simulink model "CM13_2024a_MachE_for_UA_HIL"  (R2024a)
settings: Solver=ode1  StartTime=0.0  StopTime=Inf  FixedStep=0.001  RelTol=1e-3  EnableMultiTasking=on
PreLoadFcn:
  | % if ~length(which('cmcmd')), cmenv; end
PostLoadFcn:
  | if any(exist('dsrtsu_mdlpostloadfcn', 'file') ~= 0), dsrtsu_mdlpostloadfcn('Execute', bdroot); end
InitFcn:
  | , if any(exist('rtifpga_mdlclblib', 'file') ~= 0), rtifpga_mdlclblib('Init', bdroot); end,
  | , if any(exist('dsmpb_private', 'file') ~= 0), dsmpb_private('dsmpb_mdlclblib', 'Init', bdroot); end,
values from neighbouring files (symbols this model uses):
  CoastDown =     [Run_Simulink.mat]
  limitedMCT =     [Run_Simulink.mat]
  MCT =     [Run_Simulink.mat]
  pMCT =     [Run_Simulink.mat]
  RealSimPara =     [Run_Simulink.mat]
  Ref_speed = [13 13.007895099 13.015778396 13.023649891 13.031509584 13.039357475 13.047193564 13.055017851 13.062830336 13.070631019 13.0784199 13.086196979 ... (2669 elements, 2669x1)]    [Ref_speed_and_time.mat]
  Ref_time = [0 0.01 0.02 0.03 0.04 0.05 0.06 0.07 0.08 0.09 0.1 0.11 ... (2669 elements, 2669x1)]    [Ref_speed_and_time.mat]
  US06 =     [Run_Simulink.mat]
undefined symbols (not defined in the file or in its folder): AccelCmd, ActTqLF_Nm_, ActTqLR_Nm_, ActTqRF_Nm_, ActTqRR_Nm_, BattChargeLimitMaxPwr, BattChargeLimitSocBpts, BattChargeLimitTbl, BattChrgCapcty, BattDischargeLimitSocBpts, BattDischargeLimitTbl, BattDischargeMaxPwr, BattNumCellsParallel, BattNumCellsSeries, BattOpenVoltCapBpts, BattOpenVoltTbl, BattResistSocBpts, BattResistTbl, BattResistTempBpts, BrakeMaxPrs, BrakeMaxTrq, ChassisDistCg2FrontAxle, ChassisDistCg2RearAxle, ChassisVehMass, CltchCmd, DecelCmd, DiffRatio, DiscIntNeverNeededParam, EnvGravCnst, EnvPrs, EnvTemp, FuelSpecificGrav, GearCmd, h, InitStates, lgSw, MtrEffSpdBpts, MtrEffTbl, MtrEffTrqBpts, MtrPwrMax, MtrTrqMax, planned_speed, planned_time, ref_speed, ref_time, rticanmm_blockfcn, rticanmm_initfcn, SteeringCmd, SupvsryCtrlRegenBrkCutOffTbl, SupvsryCtrlRegenSpdBpts, TestScnrioCycleNum, VEH
libraries: simulink x264, VSIGenLib x262, etargetslib x201, dsmpblib x161, CarMaker4SL x142, rtimmsu_dsrtlib x32, vehdynlibtire x24, autolibshared x19, vehdynlibsuspension x14, vehdynlibtirecommon x14, autolibutils x10, VsrLibWheel x8
(part 2 of 48)

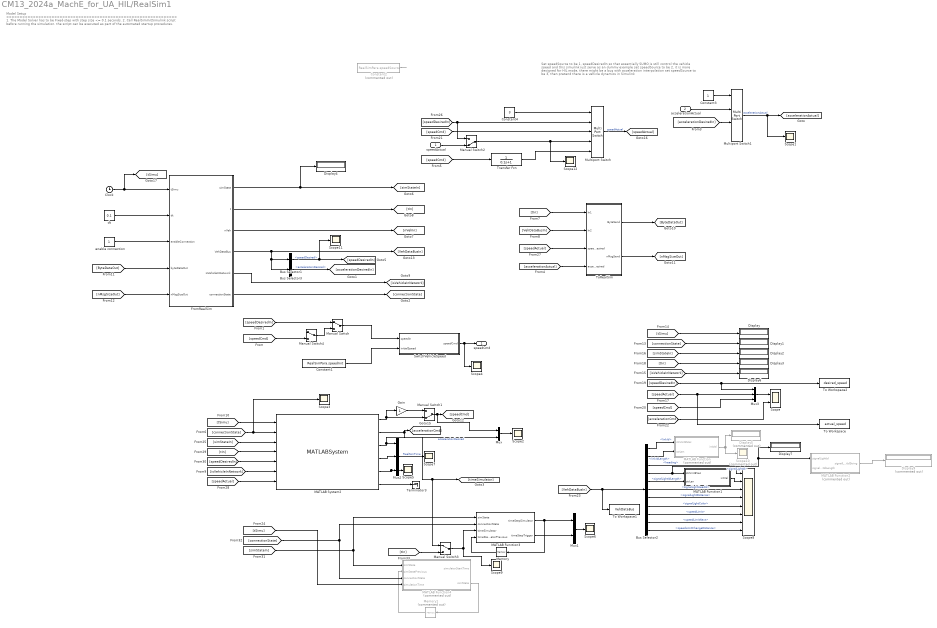
== system CM13_2024a_MachE_for_UA_HIL/RealSim1 ==
  note: Set speedSource to be 1, speedDesiredIn so that essentially SUMO is still control the vehicle speed and this simulink just serve as an dummy example
      |
      | set speedSource to be 2, it is more designed for HIL mode, there might be a bug with acceleration interpolation
      |
      | set speedSource to be 3, then pretend there is a vehicle dynamics in Simulink
  note: Model Setup
      | ================================================================
      | 1. The Model Solver has to be Fixed-step with step size <= 0.1 seconds.
      | 2. Call RealSimInitSimulink script before running the simulation. the script can be executed as part of the automated startup procedures.
  speedActual : Inport
  accelerationActual : Inport  Port=2
  Bus Selector1 : BusSelector  OutputSignals=speedDesired
  Bus Selector2 : BusSelector  OutputSignals=linkId,linkIdLength,heading,signalLightId,signalLightIdLength,signalLightHeadId,signalLightDistance,signalLightColor,speedLimit,speedLimitNext,speedLimitChangeDistance
  Bus Selector3 : BusSelector  OutputSignals=accelerationDesired
  Clock : Clock
  Constant1 : Constant  Value=RealSimPara.speedInit
  Constant2 : Constant  Commented=on  Value=RealSimPara.speedSource
  Constant3 : Constant
  Constant4 : Constant  Value=3
  Display{,1..4,6..7} (7 alike) : Display
  Display5 : Display  Commented=on
  Display9 : Display  Commented=on
  FromRealSim : Subsystem
  Gain : Gain
  MATLAB Function : MATLAB Function  Commented=on  TreatAsAtomicUnit=on
  MATLAB Function1 : MATLAB Function  TreatAsAtomicUnit=on
  MATLAB Function2 : MATLAB Function  Commented=on  TreatAsAtomicUnit=on  SystemSampleTime=0.001
  MATLAB Function3 : MATLAB Function  TreatAsAtomicUnit=on
  MATLAB Function4 : MATLAB Function  Commented=on  TreatAsAtomicUnit=on
  MATLAB System2 : MATLABSystem  System=RealSimInterpSpeed  initialSpeed=RealSimPara.speedInit  speedLookAheadHorizon=RealSimPara.tLookahead  speedUpperBound=30  smoothWindow=RealSimPara.smoothWindow  SimulateUsing=Interpreted execution
      mask Type: RealSimInterpSpeed
      mask Display:
      | disp('RealSimInterpSpeed');
      | port_label('input',1,'simulationTime');
      | port_label('input',2,'connectionState');
      | port_label('input',3,'simState');
      | port_label('input',4,'timeReceive');
      | port_label('input',5,'speedReceive');
      | port_label('input',6,'isVehicleInNetwork');
      | port_label('input',7,'speedActual');
      | port_label('output',1,'speedLookAhead');
      | port_label('output',2,'accelerationDesired');
      | port_label('output',3,'timeSimulator');
      | port_label('output',4,'timeStepSimulator');
      | port_label('output',5,'timeStepTrigger');
      | port_label('output',6,'RealSimDelay');
  Manual Switch : ManualSwitch
  Manual Switch1 : ManualSwitch  CurrentSetting=0
  Manual Switch2 : ManualSwitch  CurrentSetting=0
  Manual Switch3 : ManualSwitch
  Manual Switch4 : ManualSwitch
  Memory : Memory
  Memory1 : Memory  Commented=on
  Multiport Switch : MultiPortSwitch  Inputs=4  SaturateOnIntegerOverflow=off  InputSameDT=off
  Multiport Switch1 : MultiPortSwitch  SaturateOnIntegerOverflow=off  InputSameDT=off
  Mux : Mux  Inputs=2
  Mux1 : Mux  Inputs=2
  Mux2 : Mux  Inputs=3
  Mux3 : Mux  Inputs=3
  Scope : Scope  NumInputPorts=2
  Scope{1..7,9,11..12} (10 alike) : Scope
  Scope10 : Scope  Commented=on
  Scope8 : Scope  NumInputPorts=8
  SwitchVehicleSpeed : Subsystem
  Terminator3 : Terminator
  To Workspace : ToWorkspace  VariableName=actual_speed  SaveFormat=Timeseries  SampleTime=0.1
  To Workspace1 : ToWorkspace  VariableName=VehDataBus  SaveFormat=Timeseries  SampleTime=-1
  To Workspace2 : ToWorkspace  VariableName=desired_speed  SaveFormat=Timeseries  SampleTime=0.1
  ToRealSim : Subsystem
  Transfer Fcn : TransferFcn  Denominator=[0.1 1]
  dt : Constant  Value=0.1
  enable connection : Constant
  speedCmd : Outport
  wires:
  [speedCmd] -> Manual Switch4/2
  Manual Switch3/1 -> MATLAB Function3/3(timeSimulator), Scope9/1
  [tIn] -> Manual Switch3/2
  MATLAB Function4/2(simState) -> Memory1/1
  Memory1/1 -> MATLAB Function4/2(simStatePrevious)
  MATLAB Function3/2(timeStepTrigger) -> Mux1/2
  Mux1/1 -> Scope6/1
  Memory/1 -> MATLAB Function3/4(timeStepSimulatorPrevious)
  MATLAB Function3/1(timeStepSimulator) -> Memory/1, Mux1/1
  [simStateIn] -> MATLAB Function3/1(simState), MATLAB Function4/1("simState ")
  [connectionState] -> MATLAB Function3/2(connectionState), MATLAB Function4/3(connectionState)
  [tSimu] -> MATLAB Function4/4(simulationTime)
  Transfer Fcn/1 -> Multiport Switch/5
  [speedCmd] -> Transfer Fcn/1
  speedActual/1 -> Manual Switch2/2
  Mux/1 -> Scope2/1
  FromRealSim/6(connectionState) -> [connectionState]
  Multiport Switch1/1 -> [accelerationActual], Scope1/1  "accelerationActual"
  accelerationActual/1 -> Multiport Switch1/2
  [accelerationDesiredIn] -> Multiport Switch1/3
  Constant3/1 -> Multiport Switch1/1
  Bus Selector3/1 -> [accelerationDesiredIn]  "<accelerationDesired>"
  Manual Switch/1 -> SwitchVehicleSpeed/1(speedIn)
  SwitchVehicleSpeed/1(speedCmd) -> speedCmd/1, Scope4/1
  Constant1/1 -> SwitchVehicleSpeed/2(initialSpeed)
  [speedDesiredIn] -> Manual Switch/1
  Manual Switch4/1 -> Manual Switch/2
  Constant2/1 -> ?
  ? -> MATLAB Function2/2(signalLightIdLength)
  [simStateIn] -> Display2/1
  Mux3/1 -> Scope/1
  [isVehicleInNetwork] -> MATLAB System2/6
  Bus Selector2/3 -> Scope8/1  "<heading>"
  MATLAB Function1/1(intVal) -> Scope8/2
  ToRealSim/1(ByteSend) -> [ByteDataOut]
  [accelerationActual] -> ToRealSim/4(accelerationDesired)
  Bus Selector2/6 -> Scope8/3  "<signalLightHeadId>"
  Multiport Switch/1 -> [speedActual]  "speedActual"
  [VehDataBusIn] -> ToRealSim/2(In2)
  [accelerationCmd] -> Scope/2
  FromRealSim/5(isVehicleInNetwork) -> [isVehicleInNetwork]
  FromRealSim/2(t) -> [tIn]
  [speedActual] -> ToRealSim/3(speedDesired)
  FromRealSim/1(simState) -> [simStateIn], Display4/1
  ToRealSim/2(nMsgSend) -> [nMsgSizeOut]
  Manual Switch1/1 -> [speedCmd], Mux/1
  Constant4/1 -> Multiport Switch/1
  [speedCmd] -> Mux3/3
  [tIn] -> MATLAB System2/4
  Bus Selector2/2 -> MATLAB Function/2(strLen)  "<linkIdLength>"
  MATLAB Function2/1(signalLightIdString) -> Display9/1
  MATLAB System2/2 -> Mux/2, [accelerationCmd]  "accelerationDesired"
  [tIn] -> ToRealSim/1(In1)
  Bus Selector2/1 -> MATLAB Function/1(strUint8Vec)  "<linkId>"
  MATLAB System2/6 -> Terminator3/1
  [connectionState] -> Scope3/1, MATLAB System2/2
  Manual Switch2/1 -> Multiport Switch/4, Scope12/1
  Bus Selector2/8 -> Scope8/5  "<signalLightColor>"
  MATLAB System2/4 -> Mux2/2
  Bus Selector2/7 -> Scope8/4  "<signalLightDistance>"
  [tIn] -> Display3/1
  Clock/1 -> [tSimu], FromRealSim/1(tSimu)
  [connectionState] -> Display1/1
  [speedActual] -> Mux3/2, To Workspace/1
  FromRealSim/3(nVeh) -> [nVehIn]
  [speedActual] -> MATLAB System2/7
  [speedDesiredIn] -> Multiport Switch/2, Manual Switch2/1
  Bus Selector2/11 -> Scope8/8  "<speedLimitChangeDistance>"
  [nMsgSizeOut] -> FromRealSim/5(nMsgSizeOut)
  [speedDesiredIn] -> MATLAB System2/5
  MATLAB Function/1(intVal) -> Display5/1, Scope10/1
  enable connection/1 -> FromRealSim/3(enableConnection)
  FromRealSim/4(VehDataBus) -> Bus Selector3/1, Bus Selector1/1, [VehDataBusIn]
  Bus Selector2/10 -> Scope8/7  "<speedLimitNext>"
  dt/1 -> FromRealSim/2(dt)
  MATLAB System2/3 -> Mux2/1, Manual Switch3/1, [timeSimulator]
  Bus Selector2/4 -> MATLAB Function1/1(strUint8Vec), MATLAB Function2/1(signalLightId), Display7/1  "<signalLightId>"
  [speedDesiredIn] -> Mux3/1, To Workspace2/1
  Bus Selector2/9 -> Scope8/6  "<speedLimit>"
  Bus Selector1/1 -> [speedDesiredIn], Scope11/1  "<speedDesired>"
  Gain/1 -> Manual Switch1/1
  [tSimu] -> MATLAB System2/1
  Mux2/1 -> Scope7/1  "RealSimTime"
  [speedCmd] -> Multiport Switch/3
  MATLAB System2/1 -> Manual Switch1/2, Gain/1
  [VehDataBusIn] -> Bus Selector2/1, To Workspace1/1
  MATLAB System2/5 -> Mux2/3, Scope5/1
  [ByteDataOut] -> FromRealSim/4(byteDataOut)
  [isVehicleInNetwork] -> Display6/1
  [simStateIn] -> MATLAB System2/3
  Bus Selector2/5 -> MATLAB Function1/2(strLen)  "<signalLightIdLength>"
  [tSimu] -> Display/1

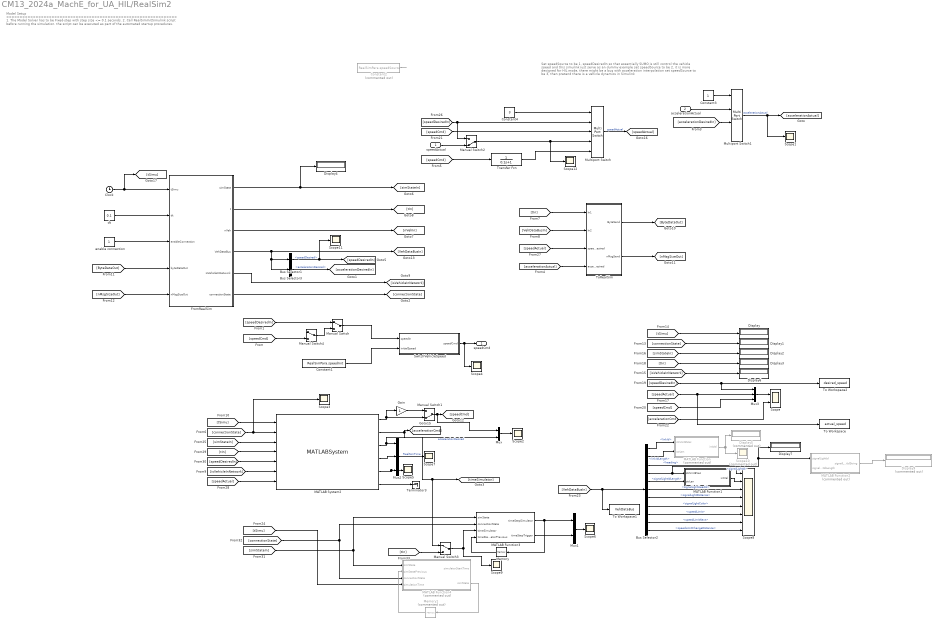
== system CM13_2024a_MachE_for_UA_HIL/RealSim2 ==
  note: Model Setup
      | ================================================================
      | 1. The Model Solver has to be Fixed-step with step size <= 0.1 seconds.
      | 2. Call RealSimInitSimulink script before running the simulation. the script can be executed as part of the automated startup procedures.
  note: Set speedSource to be 1, speedDesiredIn so that essentially SUMO is still control the vehicle speed and this simulink just serve as an dummy example
      |
      | set speedSource to be 2, it is more designed for HIL mode, there might be a bug with acceleration interpolation
      |
      | set speedSource to be 3, then pretend there is a vehicle dynamics in Simulink
  speedActual : Inport
  accelerationActual : Inport  Port=2
  Bus Selector1 : BusSelector  OutputSignals=speedDesired
  Bus Selector2 : BusSelector  OutputSignals=linkId,linkIdLength,heading,signalLightId,signalLightIdLength,signalLightHeadId,signalLightDistance,signalLightColor,speedLimit,speedLimitNext,speedLimitChangeDistance
  Bus Selector3 : BusSelector  OutputSignals=accelerationDesired
  Clock : Clock
  Constant1 : Constant  Value=RealSimPara.speedInit
  Constant2 : Constant  Commented=on  Value=RealSimPara.speedSource
  Constant3 : Constant
  Constant4 : Constant  Value=3
  Display{,1..4,6..7} (7 alike) : Display
  Display5 : Display  Commented=on
  Display9 : Display  Commented=on
  FromRealSim : Subsystem
  Gain : Gain
  MATLAB Function : MATLAB Function  Commented=on  TreatAsAtomicUnit=on
  MATLAB Function1 : MATLAB Function  TreatAsAtomicUnit=on
  MATLAB Function2 : MATLAB Function  Commented=on  TreatAsAtomicUnit=on  SystemSampleTime=0.001
  MATLAB Function3 : MATLAB Function  TreatAsAtomicUnit=on
  MATLAB Function4 : MATLAB Function  Commented=on  TreatAsAtomicUnit=on
  MATLAB System2 : MATLABSystem  System=RealSimInterpSpeed  initialSpeed=RealSimPara.speedInit  speedLookAheadHorizon=RealSimPara.tLookahead  speedUpperBound=30  smoothWindow=RealSimPara.smoothWindow  SimulateUsing=Interpreted execution
      mask Type: RealSimInterpSpeed
      mask Display:
      | disp('RealSimInterpSpeed');
      | port_label('input',1,'simulationTime');
      | port_label('input',2,'connectionState');
      | port_label('input',3,'simState');
      | port_label('input',4,'timeReceive');
      | port_label('input',5,'speedReceive');
      | port_label('input',6,'isVehicleInNetwork');
      | port_label('input',7,'speedActual');
      | port_label('output',1,'speedLookAhead');
      | port_label('output',2,'accelerationDesired');
      | port_label('output',3,'timeSimulator');
      | port_label('output',4,'timeStepSimulator');
      | port_label('output',5,'timeStepTrigger');
      | port_label('output',6,'RealSimDelay');
  Manual Switch : ManualSwitch
  Manual Switch1 : ManualSwitch  CurrentSetting=0
  Manual Switch2 : ManualSwitch  CurrentSetting=0
  Manual Switch3 : ManualSwitch
  Manual Switch4 : ManualSwitch
  Memory : Memory
  Memory1 : Memory  Commented=on
  Multiport Switch : MultiPortSwitch  Inputs=4  SaturateOnIntegerOverflow=off  InputSameDT=off
  Multiport Switch1 : MultiPortSwitch  SaturateOnIntegerOverflow=off  InputSameDT=off
  Mux : Mux  Inputs=2
  Mux1 : Mux  Inputs=2
  Mux2 : Mux  Inputs=3
  Mux3 : Mux  Inputs=3
  Scope : Scope  NumInputPorts=2
  Scope{1..7,9,11..12} (10 alike) : Scope
  Scope10 : Scope  Commented=on
  Scope8 : Scope  NumInputPorts=8
  SwitchVehicleSpeed : Subsystem
  Terminator3 : Terminator
  To Workspace : ToWorkspace  VariableName=actual_speed  SaveFormat=Timeseries  SampleTime=0.1
  To Workspace1 : ToWorkspace  VariableName=VehDataBus  SaveFormat=Timeseries  SampleTime=-1
  To Workspace2 : ToWorkspace  VariableName=desired_speed  SaveFormat=Timeseries  SampleTime=0.1
  ToRealSim : Subsystem
  Transfer Fcn : TransferFcn  Denominator=[0.1 1]
  dt : Constant  Value=0.1
  enable connection : Constant
  speedCmd : Outport
  wires:
  [tSimu] -> Display/1
  Bus Selector2/5 -> MATLAB Function1/2(strLen)  "<signalLightIdLength>"
  [simStateIn] -> MATLAB System2/3
  [isVehicleInNetwork] -> Display6/1
  [ByteDataOut] -> FromRealSim/4(byteDataOut)
  MATLAB System2/5 -> Scope5/1, Mux2/3
  [VehDataBusIn] -> To Workspace1/1, Bus Selector2/1
  MATLAB System2/1 -> Gain/1, Manual Switch1/2
  [speedCmd] -> Multiport Switch/3
  Mux2/1 -> Scope7/1  "RealSimTime"
  [tSimu] -> MATLAB System2/1
  Gain/1 -> Manual Switch1/1
  Bus Selector1/1 -> Scope11/1, [speedDesiredIn]  "<speedDesired>"
  Bus Selector2/9 -> Scope8/6  "<speedLimit>"
  [speedDesiredIn] -> To Workspace2/1, Mux3/1
  Bus Selector2/4 -> Display7/1, MATLAB Function2/1(signalLightId), MATLAB Function1/1(strUint8Vec)  "<signalLightId>"
  MATLAB System2/3 -> [timeSimulator], Manual Switch3/1, Mux2/1
  dt/1 -> FromRealSim/2(dt)
  Bus Selector2/10 -> Scope8/7  "<speedLimitNext>"
  FromRealSim/4(VehDataBus) -> [VehDataBusIn], Bus Selector1/1, Bus Selector3/1
  enable connection/1 -> FromRealSim/3(enableConnection)
  MATLAB Function/1(intVal) -> Scope10/1, Display5/1
  [speedDesiredIn] -> MATLAB System2/5
  [nMsgSizeOut] -> FromRealSim/5(nMsgSizeOut)
  Bus Selector2/11 -> Scope8/8  "<speedLimitChangeDistance>"
  [speedDesiredIn] -> Manual Switch2/1, Multiport Switch/2
  [speedActual] -> MATLAB System2/7
  FromRealSim/3(nVeh) -> [nVehIn]
  [speedActual] -> To Workspace/1, Mux3/2
  [connectionState] -> Display1/1
  Clock/1 -> FromRealSim/1(tSimu), [tSimu]
  [tIn] -> Display3/1
  Bus Selector2/7 -> Scope8/4  "<signalLightDistance>"
  MATLAB System2/4 -> Mux2/2
  Bus Selector2/8 -> Scope8/5  "<signalLightColor>"
  Manual Switch2/1 -> Scope12/1, Multiport Switch/4
  [connectionState] -> MATLAB System2/2, Scope3/1
  MATLAB System2/6 -> Terminator3/1
  Bus Selector2/1 -> MATLAB Function/1(strUint8Vec)  "<linkId>"
  [tIn] -> ToRealSim/1(In1)
  MATLAB System2/2 -> [accelerationCmd], Mux/2  "accelerationDesired"
  MATLAB Function2/1(signalLightIdString) -> Display9/1
  Bus Selector2/2 -> MATLAB Function/2(strLen)  "<linkIdLength>"
  [tIn] -> MATLAB System2/4
  [speedCmd] -> Mux3/3
  Constant4/1 -> Multiport Switch/1
  Manual Switch1/1 -> Mux/1, [speedCmd]
  ToRealSim/2(nMsgSend) -> [nMsgSizeOut]
  FromRealSim/1(simState) -> Display4/1, [simStateIn]
  [speedActual] -> ToRealSim/3(speedDesired)
  FromRealSim/2(t) -> [tIn]
  FromRealSim/5(isVehicleInNetwork) -> [isVehicleInNetwork]
  [accelerationCmd] -> Scope/2
  [VehDataBusIn] -> ToRealSim/2(In2)
  Multiport Switch/1 -> [speedActual]  "speedActual"
  Bus Selector2/6 -> Scope8/3  "<signalLightHeadId>"
  [accelerationActual] -> ToRealSim/4(accelerationDesired)
  ToRealSim/1(ByteSend) -> [ByteDataOut]
  MATLAB Function1/1(intVal) -> Scope8/2
  Bus Selector2/3 -> Scope8/1  "<heading>"
  [isVehicleInNetwork] -> MATLAB System2/6
  Mux3/1 -> Scope/1
  [simStateIn] -> Display2/1
  ? -> MATLAB Function2/2(signalLightIdLength)
  Constant2/1 -> ?
  Manual Switch4/1 -> Manual Switch/2
  [speedDesiredIn] -> Manual Switch/1
  Constant1/1 -> SwitchVehicleSpeed/2(initialSpeed)
  SwitchVehicleSpeed/1(speedCmd) -> Scope4/1, speedCmd/1
  Manual Switch/1 -> SwitchVehicleSpeed/1(speedIn)
  Bus Selector3/1 -> [accelerationDesiredIn]  "<accelerationDesired>"
  Constant3/1 -> Multiport Switch1/1
  [accelerationDesiredIn] -> Multiport Switch1/3
  accelerationActual/1 -> Multiport Switch1/2
  Multiport Switch1/1 -> Scope1/1, [accelerationActual]  "accelerationActual"
  FromRealSim/6(connectionState) -> [connectionState]
  Mux/1 -> Scope2/1
  speedActual/1 -> Manual Switch2/2
  [speedCmd] -> Transfer Fcn/1
  Transfer Fcn/1 -> Multiport Switch/5
  [tSimu] -> MATLAB Function4/4(simulationTime)
  [connectionState] -> MATLAB Function4/3(connectionState), MATLAB Function3/2(connectionState)
  [simStateIn] -> MATLAB Function4/1("simState "), MATLAB Function3/1(simState)
  MATLAB Function3/1(timeStepSimulator) -> Mux1/1, Memory/1
  Memory/1 -> MATLAB Function3/4(timeStepSimulatorPrevious)
  Mux1/1 -> Scope6/1
  MATLAB Function3/2(timeStepTrigger) -> Mux1/2
  Memory1/1 -> MATLAB Function4/2(simStatePrevious)
  MATLAB Function4/2(simState) -> Memory1/1
  [tIn] -> Manual Switch3/2
  Manual Switch3/1 -> Scope9/1, MATLAB Function3/3(timeSimulator)
  [speedCmd] -> Manual Switch4/2

== system CM13_2024a_MachE_for_UA_HIL/TCP SCALEXIO ==
  note: Receiving gas, brake, steering; or three identical speeds
  note: Sending out x, y, heading, time, and speed
  VehOutput : Inport
  comm : Inport  Port=2
  Constant2 : Constant  Value=zeros(1004,1);  OutDataTypeStr=uint8
  Data Type Conversion1 : DataTypeConversion  OutDataTypeStr=double  SaturateOnIntegerOverflow=off  RndMeth=Floor
  Data Type Conversion2 : DataTypeConversion  SaturateOnIntegerOverflow=off  RndMeth=Floor
  Data Type Conversion3 : DataTypeConversion  OutDataTypeStr=boolean  SaturateOnIntegerOverflow=off  RndMeth=Floor
  Defloater{,1..4} (5 alike) : VSIGenLib/Defloater  SystemSampleTime=-1  VariantActivationTime=update diagram  AllowFlexibleInterface=on  Latency=0  AutoFrameSizeCalculation=off
  Demux{,2..5} (5 alike) : Demux
  Demux1 : Demux  Outputs=5
  Display3 : Display
  Ethernet Setup Carla : dsmpblib/Data Inport  Priority=10000
      settings: SourceProductName=dSPACE Model Interface Package for Simulink (MIPS)
  Floater : VSIGenLib/Floater  SystemSampleTime=-1  VariantActivationTime=update diagram  AllowFlexibleInterface=on  Latency=0  AutoFrameSizeCalculation=off
  Floater1 : VSIGenLib/Floater  SystemSampleTime=-1  VariantActivationTime=update diagram  AllowFlexibleInterface=on  Latency=0  AutoFrameSizeCalculation=off
  Floater2 : VSIGenLib/Floater  SystemSampleTime=-1  VariantActivationTime=update diagram  AllowFlexibleInterface=on  Latency=0  AutoFrameSizeCalculation=off
  Mux : Mux  Inputs=21
  Mux1 : Mux  Inputs=3
  Receive [TCP Carla] : dsmpblib/Data Inport  Priority=10000
      settings: SourceProductName=dSPACE Model Interface Package for Simulink (MIPS)
  Scope1 : Scope
  Scope4 : Scope
  Selector1 : Selector  InputPortWidth=1024  IndexOptions=Index vector (dialog)  Indices=[8 7 6 5]  OutputSizes=1
  Selector2 : Selector  InputPortWidth=1024  IndexOptions=Index vector (dialog)  Indices=[12 11 10 9]  OutputSizes=1
  Selector4 : Selector  InputPortWidth=1024  IndexOptions=Index vector (dialog)  Indices=[4 3 2 1]  OutputSizes=1
  SpdAdjust : Gain  Gain=1.1414
  Status/Control_In [TCP Carla] : dsmpblib/Data Inport  Priority=10000
      settings: SourceProductName=dSPACE Model Interface Package for Simulink (MIPS)
  Status/Control_Out [TCP Carla] : dsmpblib/Data Outport  Priority=-10000
      settings: SourceProductName=dSPACE Model Interface Package for Simulink (MIPS)
  Terminator{1..5} (5 alike) : Terminator
  Transmit_In [TCP Carla] : dsmpblib/Data Inport  Priority=10000
      settings: SourceProductName=dSPACE Model Interface Package for Simulink (MIPS)
  Transmit_Out [TCP Carla] : dsmpblib/Data Outport  Priority=-10000
      settings: SourceProductName=dSPACE Model Interface Package for Simulink (MIPS)
  uint8 (unsigned 8) 4 : etargetslib/Byte Pack  datatypes={'uint8'}  byteAlign=1
  Output : Outport
  wires:
  Demux4/4 -> Mux/16
  Demux3/4 -> Mux/12
  Defloater1/1 -> Demux2/1
  Mux/1 -> Data Type Conversion2/1
  Demux4/2 -> Mux/14
  Demux3/1 -> Mux/9
  Demux/4 -> Mux/4
  Demux/1 -> Mux/1
  Demux2/4 -> Mux/8
  Demux1/3 -> Defloater2/1
  Defloater/1 -> Demux/1
  Defloater3/1 -> Demux4/1
  Demux3/3 -> Mux/11
  Demux1/2 -> Defloater1/1
  Demux2/2 -> Mux/6
  Constant2/1 -> uint8 (unsigned 8) 4/1
  Demux1/1 -> Defloater/1
  Defloater2/1 -> Demux3/1
  Demux1/4 -> Defloater3/1
  Demux3/2 -> Mux/10
  Demux/3 -> Mux/3
  Demux/2 -> Mux/2
  VehOutput/1 -> Demux1/1
  Demux2/1 -> Mux/5
  Demux4/1 -> Mux/13
  Demux2/3 -> Mux/7
  Demux4/3 -> Mux/15
  Data Type Conversion2/1 -> Transmit_Out [TCP Carla]/1
  ? -> Terminator2/1
  Transmit_In [TCP Carla]/1 -> Terminator1/1
  Receive [TCP Carla]/1 -> Selector2/1, Selector1/1, Selector4/1
  Selector4/1 -> Floater/1
  Floater/1 -> Display3/1, Mux1/1
  ? -> Terminator4/1
  Data Type Conversion3/1 -> Status/Control_Out [TCP Carla]/1
  comm/1 -> Data Type Conversion3/1
  ? -> Terminator5/1
  ? -> Terminator3/1
  Status/Control_In [TCP Carla]/1 -> Scope4/1
  Ethernet Setup Carla/1 -> Scope1/1
  Demux1/5 -> SpdAdjust/1
  Defloater4/1 -> Demux5/1
  Demux5/2 -> Mux/18
  Demux5/3 -> Mux/19
  Demux5/4 -> Mux/20
  uint8 (unsigned 8) 4/1 -> Mux/21
  Demux5/1 -> Mux/17
  SpdAdjust/1 -> Defloater4/1
  Selector1/1 -> Floater1/1
  Mux1/1 -> Data Type Conversion1/1
  Floater1/1 -> Mux1/2
  Selector2/1 -> Floater2/1
  Floater2/1 -> Mux1/3
  Data Type Conversion1/1 -> Output/1

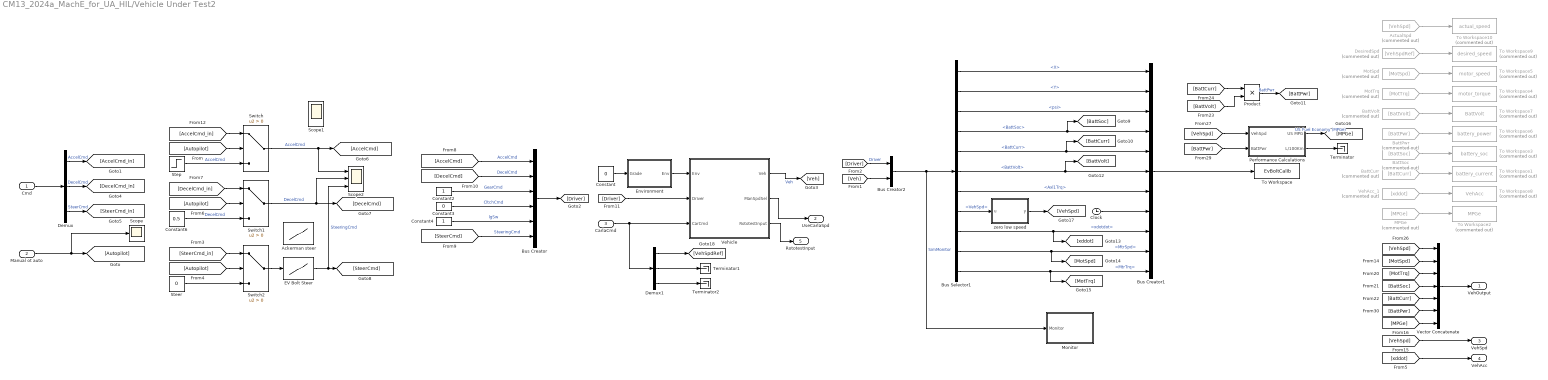
== system CM13_2024a_MachE_for_UA_HIL/Vehicle Under Test2 ==
  Cmd : Inport
  Manual ot auto : Inport  Port=2
  CarlaCmd : Inport  Port=3
  Ackerman steer : Lookup_n-D  NumberOfTableDimensions=1  BreakpointsForDimension1="[-0.446316297916244\t-0.442150786830951\t-0.437977161945005\t-0.433795286969319\t-0.429605025209166\t-0.425406239561593\t-0.421198792513030\t-0.416982546137136\t-0.412757362092861\t-0.408523101622746\t-0.404279625551461\t-0.400026794284603\t-0.395764467807732\t-0.391492505685692\t-0.387210767062193\t-0.382919110659678\t-0.378617394779480\t-0.374305477302279\t-0.369983215688866\t-0.365650466981227\t-0.361307087803951\t-0.356952934365975\t-0.352587862462675\t-0.348211727478321\t-0.343824384388886\t-0.339425687765245\t-0.335015491776758\t-0.330593650195247\t-0.326160016399396\t-0.321714443379563\t-0.317256783743034\t-0.312786889719717\t-0.308304613168298\t-0.303809805582871\t-0.299302318100048\t-0.294782001506567\t-0.290248706247410\t-0.285702282434450\t-0.281142579855627\t-0.276569447984685\t-0.271982735991464\t-0.267382292752788\t-0.262767966863931\t-0.258139606650706\t-0.253497060182174\t-0.248840175283994\t-0.244168799552432\t-0.239482780369037\t-0.234781964916014\t-0.230066200192295\t-0.225335333030331\t-0.220589210113630\t-0.215827677995039\t-0.211050583115807\t-0.206257771825433\t-0.201449090402323\t-0.196624385075265\t-0.191783502045761\t-0.186926287511198\t-0.182052587688919\t-0.177162248841170\t-0.172255117300976\t-0.167331039498945\t-0.162389861991014\t-0.157431431487183\t-0.152455594881217\t-0.147462199281363\t-0.142451092042095\t-0.137422120796894\t-0.132375133492088\t-0.127309978421782\t-0.122226504263869\t-0.117124560117169\t-0.112003995539695\t-0.106864660588066\t-0.101706405858090\t-0.0965290825265349\t-0.0913325423940914\t-0.0861166379295599\t-0.0808812223152671\t-0.0756261494937309\t-0.0703512742155897\t-0.0650564520888085\t-0.0597415396291770\t-0.0544063943121130\t-0.0490508746257825\t-0.0436748401255510\t-0.0382781514897739\t-0.0328606705769398\t-0.0274222604841732\t-0.0219627856071077\t-0.0164821117011354\t-0.0109801059440403\t-0.00545663700002112\t0\t0.00547767577609933\t0.0110656090794470\t0.0166755107772618\t0.0223075038233658\t0.0279617092740365\t0.0336382462142580\t0.0393372316825870\t0.0450587805946413\t0.0508030056652199\t0.0565700173290652\t0.0623599236602815\t0.0681728302904245\t0.0740088403252790\t0.0798680542603446\t0.0857505698950509\t0.0916564822457268\t0.0975858834573503\t0.103538862714108\t0.109515506148794\t0.115515896751090\t0.121540114274751\t0.127588235143750\t0.133660332357415\t0.139756475394610\t0.145876730117007\t0.152021158671496\t0.158189819391799\t0.164382766699339\t0.170600051003425\t0.176841718600822\t0.183107811574771\t0.189398367693541\t0.195713420308563\t0.202052998252265\t0.208417125735647\t0.214805822245717\t0.221219102442855\t0.227656976058216\t0.234119447791246\t0.240606517207442\t0.247118178636427\t0.253654421070478\t0.260215228063589\t0.266800577631217\t0.273410442150791\t0.280044788263140\t0.286703576774936\t0.293386762562311\t0.300094294475738\t0.306826115246357\t0.313582161393837\t0.320362363135953\t0.327166644299990\t0.333994922236136\t0.340847107733006\t0.347723104935443\t0.354622811264752\t0.361546117341510\t0.368492906911125\t0.375463056772267\t0.382456436708368\t0.389472909422305\t0.396512330474460\t0.403574548224288\t0.410659403775562\t0.417766730925451\t0.424896356117582\t0.432048098399246\t0.439221769382891\t0.446417173212069\t0.453634106531970\t0.460872358464695\t0.468131710589418\t0.475411936927561\t0.482712803933137\t0.490034070488372\t0.497375487904758\t0.504736799929627\t0.512117742758400\t0.519518045052588\t0.526937427963674\t0.534375605162959\t0.541832282877473\t0.549307159932028\t0.556799927797496\t0.564310270645373\t0.571837865408689\t0.579382381849329\t0.586943482631776\t0.594520823403350\t0.602114052880920\t0.609722812944144\t0.617346738735206\t0.624985458765058]"  Table="[-9.40000000000000\t-9.30000000000000\t-9.20000000000000\t-9.10000000000000\t-9\t-8.90000000000000\t-8.80000000000000\t-8.70000000000000\t-8.60000000000000\t-8.50000000000000\t-8.40000000000000\t-8.30000000000000\t-8.20000000000000\t-8.10000000000000\t-8\t-7.90000000000000\t-7.80000000000000\t-7.70000000000000\t-7.60000000000000\t-7.50000000000000\t-7.40000000000000\t-7.30000000000000\t-7.20000000000000\t-7.10000000000000\t-7\t-6.90000000000000\t-6.80000000000000\t-6.70000000000000\t-6.60000000000000\t-6.50000000000000\t-6.40000000000000\t-6.30000000000000\t-6.20000000000000\t-6.10000000000000\t-6\t-5.90000000000000\t-5.80000000000000\t-5.70000000000000\t-5.60000000000000\t-5.50000000000000\t-5.40000000000000\t-5.30000000000000\t-5.20000000000000\t-5.10000000000000\t-5\t-4.90000000000000\t-4.80000000000000\t-4.70000000000000\t-4.60000000000000\t-4.50000000000000\t-4.40000000000000\t-4.30000000000000\t-4.20000000000000\t-4.10000000000000\t-4\t-3.90000000000000\t-3.80000000000000\t-3.70000000000000\t-3.60000000000000\t-3.50000000000000\t-3.40000000000000\t-3.30000000000000\t-3.20000000000000\t-3.10000000000000\t-3\t-2.90000000000000\t-2.80000000000000\t-2.70000000000000\t-2.60000000000000\t-2.50000000000000\t-2.40000000000000\t-2.30000000000000\t-2.20000000000000\t-2.10000000000000\t-2\t-1.90000000000000\t-1.80000000000000\t-1.70000000000000\t-1.60000000000000\t-1.50000000000000\t-1.40000000000000\t-1.30000000000000\t-1.20000000000000\t-1.10000000000000\t-1\t-0.900000000000000\t-0.800000000000000\t-0.700000000000000\t-0.600000000000000\t-0.500000000000000\t-0.400000000000000\t-0.300000000000000\t-0.200000000000000\t-0.100000000000000\t0\t0.100000000000000\t0.200000000000000\t0.300000000000000\t0.400000000000000\t0.500000000000000\t0.600000000000000\t0.700000000000000\t0.800000000000000\t0.900000000000000\t1\t1.10000000000000\t1.20000000000000\t1.30000000000000\t1.40000000000000\t1.50000000000000\t1.60000000000000\t1.70000000000000\t1.80000000000000\t1.90000000000000\t2\t2.10000000000000\t2.20000000000000\t2.30000000000000\t2.40000000000000\t2.50000000000000\t2.60000000000000\t2.70000000000000\t2.80000000000000\t2.90000000000000\t3\t3.10000000000000\t3.20000000000000\t3.30000000000000\t3.40000000000000\t3.50000000000000\t3.60000000000000\t3.70000000000000\t3.80000000000000\t3.90000000000000\t4\t4.10000000000000\t4.20000000000000\t4.30000000000000\t4.40000000000000\t4.50000000000000\t4.60000000000000\t4.70000000000000\t4.80000000000000\t4.90000000000000\t5\t5.10000000000000\t5.20000000000000\t5.30000000000000\t5.40000000000000\t5.50000000000000\t5.60000000000000\t5.70000000000000\t5.80000000000000\t5.90000000000000\t6\t6.10000000000000\t6.20000000000000\t6.30000000000000\t6.40000000000000\t6.50000000000000\t6.60000000000000\t6.70000000000000\t6.80000000000000\t6.90000000000000\t7\t7.10000000000000\t7.20000000000000\t7.30000000000000\t7.40000000000000\t7.50000000000000\t7.60000000000000\t7.70000000000000\t7.80000000000000\t7.90000000000000\t8\t8.10000000000000\t8.20000000000000\t8.30000000000000\t8.40000000000000\t8.50000000000000\t8.60000000000000\t8.70000000000000\t8.80000000000000\t8.90000000000000\t9\t9.10000000000000\t9.20000000000000\t9.30000000000000\t9.40000000000000]"  InternalRulePriority=Speed  RndMeth=Simplest
  ActualSpd : From  Commented=on  GotoTag=VehSpd
  BattCurr : From  Commented=on  GotoTag=BattCurr
  BattPwr : From  Commented=on  GotoTag=BattPwr
  BattSoc : From  Commented=on  GotoTag=BattSoc
  BattVolt : From  Commented=on  GotoTag=BattVolt
  Bus Creator : BusCreator  Inputs=AccelCmd,DecelCmd,GearCmd,CltchCmd,lgSw,SteeringCmd
  Bus Creator1 : BusCreator  Inputs=11
  Bus Creator2 : BusCreator  Inputs=2
  Bus Selector1 : BusSelector  OutputSignals=Veh.Chassis.X,Veh.Chassis.Y,Veh.Chassis.psi,Veh.Batt.BattSoc,Veh.Batt.BattCurr,Veh.Batt.BattVolt,Veh.Diff.Axl1.Axl1Trq,Veh.Chassis.VehSpd,Veh.Chassis.xdotdot,Veh.Mtr.MtrSpd,Veh.Mtr.MtrTrq
  Clock : Clock
  Constant : Constant  Value=0
  Constant2 : Constant
  Constant3 : Constant  Value=0
  Constant4 : Constant
  Constant6 : Constant  Value=0.5  SampleTime=-1
  Demux : Demux  Outputs=3
  Demux1 : Demux  Outputs=3
  DesiredSpd : From  Commented=on  GotoTag=VehSpdRef
  EV Bolt Steer : Lookup_n-D  NumberOfTableDimensions=1  BreakpointsForDimension1="[-0.541571931581492\t-0.535619550629112\t-0.529667169676731\t-0.523714788724350\t-0.517762407771969\t-0.511810026819588\t-0.505857645867207\t-0.499905264914826\t-0.493952883962445\t-0.488000503010064\t-0.482048122057683\t-0.476095741105302\t-0.470143360152921\t-0.464190979200541\t-0.458238598248160\t-0.452286217295779\t-0.446333836343398\t-0.440381455391017\t-0.434429074438636\t-0.428476693486255\t-0.422524312533874\t-0.416571931581493\t-0.410619550629112\t-0.404667169676731\t-0.398714788724350\t-0.392762407771969\t-0.386810026819588\t-0.380857645867207\t-0.374905264914826\t-0.368952883962445\t-0.363000503010064\t-0.357048122057683\t-0.351095741105302\t-0.345143360152921\t-0.339190979200541\t-0.333238598248160\t-0.327286217295779\t-0.321333836343398\t-0.315381455391017\t-0.309429074438636\t-0.303476693486255\t-0.297524312533874\t-0.291571931581493\t-0.285619550629112\t-0.279667169676731\t-0.273714788724350\t-0.267762407771969\t-0.261810026819588\t-0.255857645867207\t-0.249905264914826\t-0.243952883962445\t-0.238000503010065\t-0.232048122057684\t-0.226095741105303\t-0.220143360152922\t-0.214190979200541\t-0.208238598248160\t-0.202286217295779\t-0.196333836343398\t-0.190381455391017\t-0.184429074438636\t-0.178476693486255\t-0.172524312533874\t-0.166571931581493\t-0.160619550629112\t-0.154667169676731\t-0.148714788724350\t-0.142762407771969\t-0.136810026819588\t-0.130857645867207\t-0.124905264914826\t-0.118952883962445\t-0.113000503010064\t-0.107048122057683\t-0.101095741105303\t-0.0951433601529216\t-0.0891909792005406\t-0.0832385982481596\t-0.0772862172957787\t-0.0713338363433977\t-0.0653814553910168\t-0.0594290744386358\t-0.0534766934862548\t-0.0475243125338739\t-0.0415719315814929\t-0.0356195506291120\t-0.0296671696767310\t-0.0237147887243500\t-0.0177624077719691\t-0.0118100268195881\t-0.00585764586720720\t0\t0.00585764586720720\t0.0118100268195881\t0.0177624077719691\t0.0237147887243500\t0.0296671696767310\t0.0356195506291120\t0.0415719315814929\t0.0475243125338739\t0.0534766934862548\t0.0594290744386358\t0.0653814553910168\t0.0713338363433977\t0.0772862172957787\t0.0832385982481596\t0.0891909792005406\t0.0951433601529216\t0.101095741105303\t0.107048122057683\t0.113000503010064\t0.118952883962445\t0.124905264914826\t0.130857645867207\t0.136810026819588\t0.142762407771969\t0.148714788724350\t0.154667169676731\t0.160619550629112\t0.166571931581493\t0.172524312533874\t0.178476693486255\t0.184429074438636\t0.190381455391017\t0.196333836343398\t0.202286217295779\t0.208238598248160\t0.214190979200541\t0.220143360152922\t0.226095741105303\t0.232048122057684\t0.238000503010065\t0.243952883962445\t0.249905264914826\t0.255857645867207\t0.261810026819588\t0.267762407771969\t0.273714788724350\t0.279667169676731\t0.285619550629112\t0.291571931581493\t0.297524312533874\t0.303476693486255\t0.309429074438636\t0.315381455391017\t0.321333836343398\t0.327286217295779\t0.333238598248160\t0.339190979200541\t0.345143360152921\t0.351095741105302\t0.357048122057683\t0.363000503010064\t0.368952883962445\t0.374905264914826\t0.380857645867207\t0.386810026819588\t0.392762407771969\t0.398714788724350\t0.404667169676731\t0.410619550629112\t0.416571931581493\t0.422524312533874\t0.428476693486255\t0.434429074438636\t0.440381455391017\t0.446333836343398\t0.452286217295779\t0.458238598248160\t0.464190979200541\t0.470143360152921\t0.476095741105302\t0.482048122057683\t0.488000503010064\t0.493952883962445\t0.499905264914826\t0.505857645867207\t0.511810026819588\t0.517762407771969\t0.523714788724350\t0.529667169676731\t0.535619550629112\t0.541571931581492]"  Table="[-9.10000000000000\t-9\t-8.90000000000000\t-8.80000000000000\t-8.70000000000000\t-8.60000000000000\t-8.50000000000000\t-8.40000000000000\t-8.30000000000000\t-8.20000000000000\t-8.10000000000000\t-8\t-7.90000000000000\t-7.80000000000000\t-7.70000000000000\t-7.60000000000000\t-7.50000000000000\t-7.40000000000000\t-7.30000000000000\t-7.20000000000000\t-7.10000000000000\t-7\t-6.90000000000000\t-6.80000000000000\t-6.70000000000000\t-6.60000000000000\t-6.50000000000000\t-6.40000000000000\t-6.30000000000000\t-6.20000000000000\t-6.10000000000000\t-6\t-5.90000000000000\t-5.80000000000000\t-5.70000000000000\t-5.60000000000000\t-5.50000000000000\t-5.40000000000000\t-5.30000000000000\t-5.20000000000000\t-5.10000000000000\t-5\t-4.90000000000000\t-4.80000000000000\t-4.70000000000000\t-4.60000000000000\t-4.50000000000000\t-4.40000000000000\t-4.30000000000000\t-4.20000000000000\t-4.10000000000000\t-4\t-3.90000000000000\t-3.80000000000000\t-3.70000000000000\t-3.60000000000000\t-3.50000000000000\t-3.40000000000000\t-3.30000000000000\t-3.20000000000000\t-3.10000000000000\t-3\t-2.90000000000000\t-2.80000000000000\t-2.70000000000000\t-2.60000000000000\t-2.50000000000000\t-2.40000000000000\t-2.30000000000000\t-2.20000000000000\t-2.10000000000000\t-2\t-1.90000000000000\t-1.80000000000000\t-1.70000000000000\t-1.60000000000000\t-1.50000000000000\t-1.40000000000000\t-1.30000000000000\t-1.20000000000000\t-1.10000000000000\t-1\t-0.900000000000000\t-0.800000000000000\t-0.700000000000000\t-0.600000000000000\t-0.500000000000000\t-0.400000000000000\t-0.300000000000000\t-0.200000000000000\t-0.100000000000000\t0\t0.100000000000000\t0.200000000000000\t0.300000000000000\t0.400000000000000\t0.500000000000000\t0.600000000000000\t0.700000000000000\t0.800000000000000\t0.900000000000000\t1\t1.10000000000000\t1.20000000000000\t1.30000000000000\t1.40000000000000\t1.50000000000000\t1.60000000000000\t1.70000000000000\t1.80000000000000\t1.90000000000000\t2\t2.10000000000000\t2.20000000000000\t2.30000000000000\t2.40000000000000\t2.50000000000000\t2.60000000000000\t2.70000000000000\t2.80000000000000\t2.90000000000000\t3\t3.10000000000000\t3.20000000000000\t3.30000000000000\t3.40000000000000\t3.50000000000000\t3.60000000000000\t3.70000000000000\t3.80000000000000\t3.90000000000000\t4\t4.10000000000000\t4.20000000000000\t4.30000000000000\t4.40000000000000\t4.50000000000000\t4.60000000000000\t4.70000000000000\t4.80000000000000\t4.90000000000000\t5\t5.10000000000000\t5.20000000000000\t5.30000000000000\t5.40000000000000\t5.50000000000000\t5.60000000000000\t5.70000000000000\t5.80000000000000\t5.90000000000000\t6\t6.10000000000000\t6.20000000000000\t6.30000000000000\t6.40000000000000\t6.50000000000000\t6.60000000000000\t6.70000000000000\t6.80000000000000\t6.90000000000000\t7\t7.10000000000000\t7.20000000000000\t7.30000000000000\t7.40000000000000\t7.50000000000000\t7.60000000000000\t7.70000000000000\t7.80000000000000\t7.90000000000000\t8\t8.10000000000000\t8.20000000000000\t8.30000000000000\t8.40000000000000\t8.50000000000000\t8.60000000000000\t8.70000000000000\t8.80000000000000\t8.90000000000000\t9\t9.10000000000000]"  InternalRulePriority=Speed  RndMeth=Simplest
  Environment : Subsystem
  MPGe : From  Commented=on  GotoTag=MPGe
  Monitor : Subsystem
  MotSpd : From  Commented=on  GotoTag=MotSpd
  MotTrq : From  Commented=on  GotoTag=MotTrq
  Performance Calculations : Subsystem
  Product : Product
  Scope : Scope
  Scope1 : Scope  NumInputPorts=3
  Scope2 : Scope  NumInputPorts=3
  Steer : Constant  Value=0
  Step : Step  Time=5  After=0
  Switch : Switch  Criteria=u2 > Threshold  SaturateOnIntegerOverflow=off  InputSameDT=off
  Switch1 : Switch  Criteria=u2 > Threshold  SaturateOnIntegerOverflow=off  InputSameDT=off
  Switch2 : Switch  Criteria=u2 > Threshold  SaturateOnIntegerOverflow=off  InputSameDT=off
  Terminator : Terminator
  Terminator1 : Terminator
  Terminator2 : Terminator
  To Workspace : ToWorkspace  VariableName=EvBoltCalib  SaveFormat=Structure With Time  SampleTime=-1
  To Workspace1 : ToWorkspace  Commented=on  VariableName=battery_current  SaveFormat=Timeseries  SampleTime=0.1
  To Workspace10 : ToWorkspace  Commented=on  VariableName=actual_speed  SaveFormat=Timeseries  SampleTime=0.1
  To Workspace2 : ToWorkspace  Commented=on  VariableName=MPGe  SaveFormat=Timeseries  SampleTime=0.1
  To Workspace3 : ToWorkspace  Commented=on  VariableName=battery_soc  SaveFormat=Timeseries  SampleTime=0.1
  To Workspace4 : ToWorkspace  Commented=on  VariableName=motor_torque  SaveFormat=Timeseries  SampleTime=0.1
  To Workspace5 : ToWorkspace  Commented=on  VariableName=motor_speed  SaveFormat=Timeseries  SampleTime=0.1
  To Workspace6 : ToWorkspace  Commented=on  VariableName=battery_power  SaveFormat=Timeseries  SampleTime=0.1
  To Workspace7 : ToWorkspace  Commented=on  VariableName=BattVolt  SaveFormat=Timeseries  SampleTime=0.1
  To Workspace8 : ToWorkspace  Commented=on  VariableName=VehAcc  SaveFormat=Timeseries  SampleTime=0.1
  To Workspace9 : ToWorkspace  Commented=on  VariableName=desired_speed  SaveFormat=Timeseries  SampleTime=0.1
  Vector Concatenate : Concatenate  NumInputs=7
  VehAcc_1 : From  Commented=on  GotoTag=xddot
  Vehicle : Subsystem
  zero low speed : MATLAB Function  TreatAsAtomicUnit=on
  VehOutput : Outport
  UseCarlaSpd : Outport  Port=2
  VehSpd : Outport  Port=3
  VehAcc : Outport  Port=4
  RototestInput : Outport  Port=5
  wires:
  Bus Creator2/1 -> Bus Selector1/1, Monitor/1(Monitor)  "SimMonitor"
  [Driver] -> Bus Creator2/1  "Driver"
  Constant3/1 -> Bus Creator/4  "CltchCmd"
  Cmd/1 -> Demux/1
  Bus Creator/1 -> [Driver]
  Vehicle/1(Veh) -> [Veh]  "Veh"
  Environment/1(Env) -> Vehicle/1(Env)
  Constant/1 -> Environment/1(Grade)
  Constant4/1 -> Bus Creator/5  "lgSw"
  Bus Creator1/1 -> To Workspace/1
  Constant2/1 -> Bus Creator/3  "GearCmd"
  Vector Concatenate/1 -> VehOutput/1
  Clock/1 -> Bus Creator1/8
  Bus Selector1/1 -> Bus Creator1/1  "<X>"
  Bus Selector1/2 -> Bus Creator1/2  "<Y>"
  Bus Selector1/3 -> Bus Creator1/3  "<psi>"
  Bus Selector1/4 -> Bus Creator1/4, [BattSoc]  "<BattSoc>"
  Bus Selector1/5 -> Bus Creator1/5, [BattCurr]  "<BattCurr>"
  Bus Selector1/6 -> [BattVolt], Bus Creator1/6  "<BattVolt>"
  Bus Selector1/7 -> Bus Creator1/7  "<Axl1Trq>"
  Bus Selector1/8 -> zero low speed/1(u)  "<VehSpd>"
  [SteerCmd] -> Bus Creator/6  "SteeringCmd"
  Switch2/1 -> EV Bolt Steer/1
  Switch/1 -> Scope2/1, [AccelCmd]  "AccelCmd"
  Switch1/1 -> Scope2/2, [DecelCmd]  "DecelCmd"
  Manual ot auto/1 -> Scope/1, [Autopilot]
  [Autopilot] -> Switch/2
  Step/1 -> Switch/3  "AccelCmd"
  Demux/1 -> [AccelCmd_in]  "AccelCmd"
  Constant6/1 -> Switch1/3  "DecelCmd"
  Demux/2 -> [DecelCmd_in]  "DecelCmd"
  Steer/1 -> Switch2/3
  Demux/3 -> [SteerCmd_in]  "SteerCmd"
  CarlaCmd/1 -> Demux1/1, Vehicle/3(CarCmd)
  Vehicle/2(ManSpdSel) -> UseCarlaSpd/1
  [Veh] -> Bus Creator2/2
  Bus Selector1/9 -> Bus Creator1/9, [xddot]  "<xdotdot>"
  [AccelCmd_in] -> Switch/1
  [Autopilot] -> Switch2/2
  [SteerCmd_in] -> Switch2/1
  [Autopilot] -> Switch1/2
  [DecelCmd_in] -> Switch1/1
  [AccelCmd] -> Bus Creator/1  "AccelCmd"
  EV Bolt Steer/1 -> Scope2/3, [SteerCmd]  "SteeringCmd"
  [DecelCmd] -> Bus Creator/2  "DecelCmd"
  [Driver] -> Vehicle/2(Driver)
  Bus Selector1/10 -> Bus Creator1/10, [MotSpd]  "<MtrSpd>"
  Bus Selector1/11 -> Bus Creator1/11, [MotTrq]  "<MtrTrq>"
  Product/1 -> [BattPwr]  "BattPwr"
  Performance Calculations/1(US MPG) -> [MPGe]  "US Fuel Economy (MPGe)"
  Performance Calculations/2(L/100Km) -> Terminator/1
  [MotSpd] -> Vector Concatenate/2
  [MotTrq] -> Vector Concatenate/3
  [BattSoc] -> Vector Concatenate/4
  [BattCurr] -> Vector Concatenate/5
  [BattVolt] -> Product/2
  [BattCurr] -> Product/1
  VehAcc_1/1 -> To Workspace8/1
  [VehSpd] -> Vector Concatenate/1
  [VehSpd] -> Performance Calculations/1(VehSpd)
  BattPwr/1 -> To Workspace6/1
  [BattPwr] -> Performance Calculations/2(BattPwr)
  [BattPwr] -> Vector Concatenate/6
  BattSoc/1 -> To Workspace3/1
  BattCurr/1 -> To Workspace1/1
  MotSpd/1 -> To Workspace5/1
  MotTrq/1 -> To Workspace4/1
  [xddot] -> VehAcc/1
  MPGe/1 -> To Workspace2/1
  [VehSpd] -> VehSpd/1
  [MPGe] -> Vector Concatenate/7
  BattVolt/1 -> To Workspace7/1
  DesiredSpd/1 -> To Workspace9/1
  Demux1/1 -> [VehSpdRef]
  Demux1/2 -> Terminator1/1
  Demux1/3 -> Terminator2/1
  ActualSpd/1 -> To Workspace10/1
  Vehicle/3(RototestInput) -> RototestInput/1
  zero low speed/1(y) -> [VehSpd]
